simulink model "input_signal_test_plot"  (R2013a)
settings: Solver=VariableStepDiscrete  StartTime=0.0  StopTime=10.0  MaxStep=0.01  RelTol=1e-3
undefined symbols (not defined in the file or in its folder): da, dp, ds, r
settings Model: Creator=Vittorio  LastModifiedBy=Vittorio
settings OptimizationCC: ExpressionDepthLimit=2147483647
settings DebuggingCC: UnderspecifiedInitializationDetection=Simplified
settings GRTTargetCC: CombineOutputUpdateFcns=off  GRTInterface=on

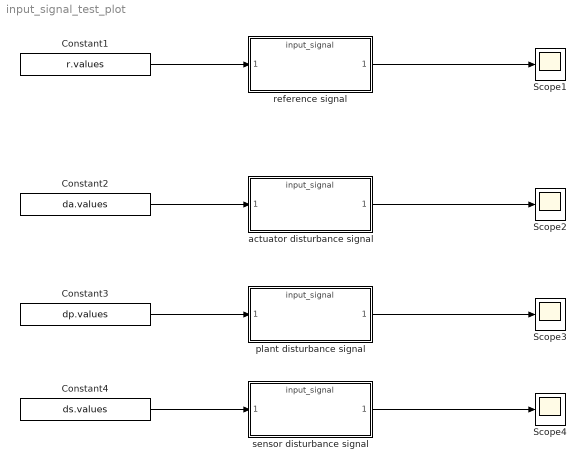
== system input_signal_test_plot ==
  Constant1 : Constant  Value=r.values  OutDataTypeStr=Bus: slBus1
  Constant2 : Constant  Value=da.values  OutDataTypeStr=Bus: slBus1
  Constant3 : Constant  Value=dp.values  OutDataTypeStr=Bus: slBus1
  Constant4 : Constant  Value=ds.values  OutDataTypeStr=Bus: slBus1
  Scope{1..4} (4 alike) : Scope
      Scope3 settings: SaveName=ScopeData2
      Scope4 settings: SaveName=ScopeData3
  actuator disturbance signal : ModelReference  ModelNameDialog=input_signal.slx  ModelReferenceVersion=1.21  CopyOfModelName=input_signal.slx  DefaultDataLogging=off
  plant disturbance signal : ModelReference  ModelNameDialog=input_signal.slx  ModelReferenceVersion=1.21  CopyOfModelName=input_signal.slx  DefaultDataLogging=off
  reference signal : ModelReference  ModelNameDialog=input_signal.slx  ModelReferenceVersion=1.21  CopyOfModelName=input_signal.slx  DefaultDataLogging=off
  sensor disturbance signal : ModelReference  ModelNameDialog=input_signal.slx  ModelReferenceVersion=1.21  CopyOfModelName=input_signal.slx  DefaultDataLogging=off
  wires:
  reference signal/1 -> Scope1/1
  Constant1/1 -> reference signal/1
  actuator disturbance signal/1 -> Scope2/1
  Constant2/1 -> actuator disturbance signal/1
  plant disturbance signal/1 -> Scope3/1
  Constant3/1 -> plant disturbance signal/1
  sensor disturbance signal/1 -> Scope4/1
  Constant4/1 -> sensor disturbance signal/1
